simulink model "mpc_preview"  (Simulink 6.0)
settings: Solver=ode5  SolverMode=SingleTasking  StartTime=0  StopTime=Tstop  RelTol=1e-3
values from neighbouring files (symbols this model uses):
  A = [-.0151 -60.5651 0 -32.174 ... (first row only)    [afti16.m]    (also in misoss.m = sys.a)
  B = [-2.516 -13.136 ... (first row only)    [afti16.m]    (also in misoss.m = sys.b)
  C = [0 1 0 0 ... (first row only)    [afti16.m]    (also in misoss.m = sys.c)
  D = [0 0 ... (first row only)    [afti16.m]    (also in misoss.m = sys.d)
  Ts = .05    (= 0.05)    [afti16.m]    (also in misoss.m = 0.2; mpcrtwdemo.m = 0.2)
libraries: mpclib x1
settings Model: Creator=jowen  LastModifiedBy=jowen  ExtModeTrigMode=oneshot  ExtModeArmWhenConnect=off
settings DataIOCC: LimitDataPoints=off  SignalLoggingName=sigsOut
settings OptimizationCC: BooleanDataType=off
settings DebuggingCC: CheckExecutionContextPreStartOutputMsg=on  CheckExecutionContextRuntimeOutputMsg=on  SolverPrmCheckMsg=none  IntegerOverflowMsg=none
settings HardwareCC: TargetUnknown=on
settings SFSimCC: SFSimApplyToAllLibs=on  SFSimBuildMode=Incremental

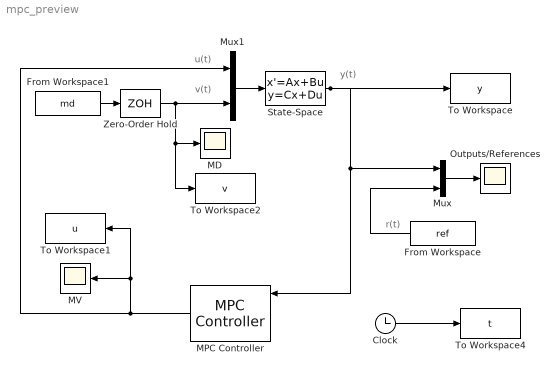
== system mpc_preview ==
  note: u(t)
  note: y(t)
  note: r(t)
  note: v(t)
  Clock : Clock
      settings: Decimation=10
  From Workspace : FromWorkspace  Orientation=left  VariableName=ref  SampleTime=0  OutputAfterFinalValue=Holding final value
  From Workspace1 : FromWorkspace  VariableName=md  SampleTime=0  OutputAfterFinalValue=Holding final value
  MD : Scope
      settings: TimeRange=30  YMin=-1  YMax=0  DataFormat=Structure
  MPC Controller : mpclib/MPC Controller  Orientation=left  mpcobj=mpc1  n_mv=0  x0=[]  ref_from_ws=on  ref_signal_name=ref  ref_preview=on  md_from_ws=on  md_signal_name=md  md_preview=on  from_project=off  md_inport=on  project_file=MPCtask.mat
  MV : Scope
      settings: TimeRange=30  YMin=-0.5  YMax=2.5  DataFormat=Structure
  Mux : Mux  Inputs=2
  Mux1 : Mux  Inputs=2
  Outputs/References : Scope
      settings: TimeRange=30  YMin=-0.5  YMax=1.5  DataFormat=Structure
  State-Space : StateSpace  A=A  B=B  C=C  D=D
  To Workspace : ToWorkspace  VariableName=y  SampleTime=-1  SaveFormat=Array
      settings: MaxDataPoints=Inf
  To Workspace1 : ToWorkspace  VariableName=u  SampleTime=-1  SaveFormat=Array
      settings: MaxDataPoints=Inf
  To Workspace2 : ToWorkspace  VariableName=v  SampleTime=-1  SaveFormat=Array
      settings: MaxDataPoints=Inf
  To Workspace4 : ToWorkspace  VariableName=t  SampleTime=-1  SaveFormat=Array
      settings: MaxDataPoints=Inf
  Zero-Order Hold : ZeroOrderHold  SampleTime=Ts
  wires:
  Mux1/1 -> State-Space/1
  Mux/1 -> Outputs/References/1
  From Workspace/1 -> Mux/2
  MPC Controller/1 -> Mux1/1, To Workspace1/1, MV/1
  Clock/1 -> To Workspace4/1
  State-Space/1 -> To Workspace/1, Mux/1, MPC Controller/1
  From Workspace1/1 -> Zero-Order Hold/1
  Zero-Order Hold/1 -> Mux1/2, MD/1, To Workspace2/1
